simulink model "regenerative_brk_27_08"  (R2023a)
settings: Solver=VariableStepAuto  StartTime=0.0  StopTime=10.0  RelTol=1e-3
undefined symbols (not defined in the file): Ion, Lithium, Regen_brkg_Bat_SOC_lowr_tshld, Regen_brkg_Bat_SOC_upp_tshld, Regen_brkg_Bat_temp_lowr_tshld, Regen_brkg_Bat_temp_uppr_tshld, Regen_brkg_Bat_vtg_lowr_tshld, Regen_brkg_Bat_vtg_uppr_tshld, Regen_brkg_Brk_Frce_uppr_tshld, Regen_brkg_hall_sensr_vtg_lowr_tshld, Regen_brkg_Inverter_crnt_uppr_tshld, Regen_brkg_Motor_crnt_uppr_tshld, Regen_brkg_Motor_OFF_tshld, Regen_brkg_Motor_ON_tshld, Regen_brkg_Motor_spd_tshld, Regen_brkg_Motor_temp_uppr_tshld, Regen_brkg_spr_cap_temp_uppr_tshld, Regen_brkg_spr_cap_vtg_uppr_tshld, Regen_brkg_system_crnt_lowr_tshld, Regen_brkg_system_crnt_uppr_tshld, Regen_brkg_vhcl_ignition_status_OFF, Regen_brkg_vhcl_ignition_status_ON, Regen_brkg_vhcl_spd_lowr_tshld
libraries: simulink x8, spsMosfetLib x6, spsVoltageMeasurementLib x3, spsBatteryLib x1, spsPermanentMagnetSynchronousMachineLib x1, slpidlib x1
settings Model: DataDictionary=RGB_DataDictionary.sldd  Creator=lenovo  LastModifiedBy=Dell

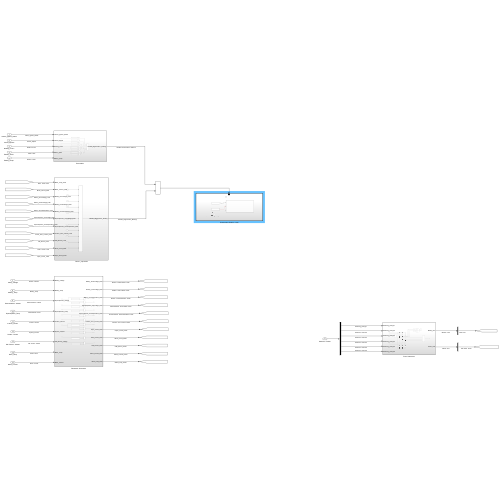
[thumbnail: Simulink's stored preview of the top-level diagram]
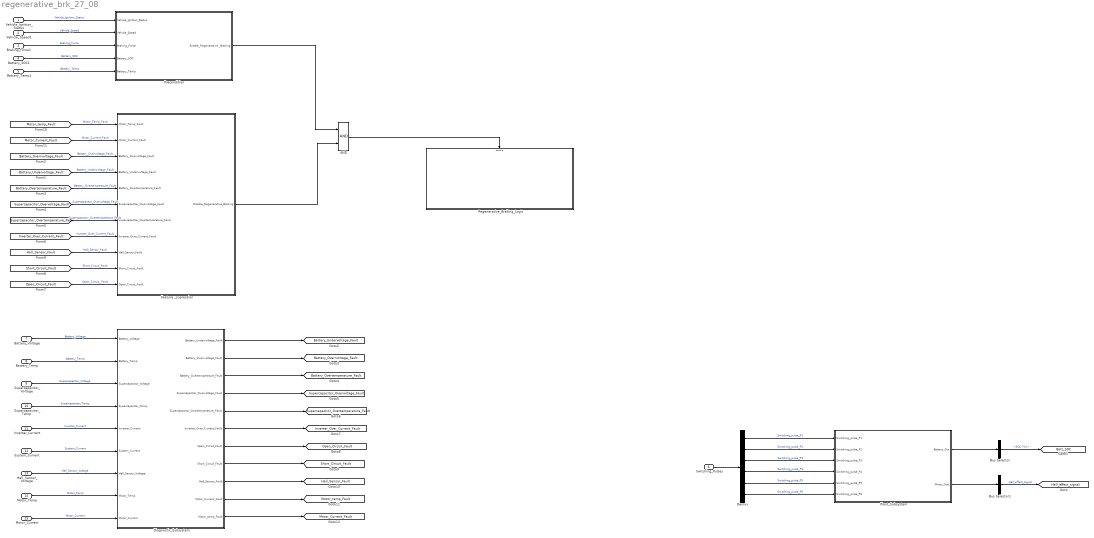
== system regenerative_brk_27_08 ==
  Vehicle_Ignition_Status : Inport
  Vehicle_Speed1 : Inport  Port=2
  Braking_Force1 : Inport  Port=3
  Battery_SOC1 : Inport  Port=4
  Battery_Temp1 : Inport  Port=5
  Switching_Pulses : Inport  Port=6
  Battery_Voltage : Inport  Port=7
  Battery_Temp : Inport  Port=8
  Supercapacitor_Voltage : Inport  Port=9
  Supercapacitor_Temp : Inport  Port=10
  Inverter_Current : Inport  Port=11
  System_Current : Inport  Port=12
  Hall_Sensor_Voltage : Inport  Port=13
  Motor_Temp : Inport  Port=14
  Motor_Current : Inport  Port=15
  AND : Logic  AllPortsSameDT=off  OutDataTypeStr=boolean
  Bus Selector : BusSelector  OutputSignals=SOC (%)
  Bus Selector1 : BusSelector  OutputSignals=Hall effect signal h_a,Hall effect signal h_b,Hall effect signal h_c  OutputAsBus=on
  Demux : Demux  Outputs=6
  Diagnostic_Subsystem : Subsystem
  Feature _supression : Subsystem
  Plant_Subsystem : Subsystem
  Precondition : Subsystem
  Regenerative_Braking_Logic : Subsystem  TreatAsAtomicUnit=on
  tag scope: Batt_SOC=global, Battery_Overrvoltage_Fault=global, Battery_Overtemperature_Fault=global, Battery_Undervoltage_Fault=global, Hall_Sensor_Fault=global, Hall_effect_signal=global, Inverter_Over_Current_Fault=global, Motor_Current_Fault=global, Motor_temp_Fault=global, Open_Circuit_Fault=global, Short_Circuit_Fault=global, Supercapacitor_Overtemperature_Fault=global, Supercapacitor_Overvoltage_Fault=global
  wires:
  [Motor_temp_Fault] -> Feature _supression/1(Motor_Temp_Fault)  "Motor_Temp_Fault"
  Feature _supression/1(Disable_Regenerative_Braking) -> AND/2
  Battery_Temp1/1 -> Precondition/5(Battery_Temp)  "Battery_Temp"
  Vehicle_Speed1/1 -> Precondition/2(Vehicle_Speed)  "Vehicle_Speed"
  Precondition/1(Enable_Regenerative _Braking) -> AND/1
  Braking_Force1/1 -> Precondition/3(Braking_Force)  "Braking_Force"
  Vehicle_Ignition_Status/1 -> Precondition/1(Vehicle_Ignition_Status)  "Vehicle_Ignition_Status"
  Battery_SOC1/1 -> Precondition/4(Battery_SOC)  "Battery_SOC"
  [Inverter_Over_Current_Fault] -> Feature _supression/8("Inverter_Over_Current_Fault ")  "Inverter_Over_Current_Fault"
  [Short_Circuit_Fault] -> Feature _supression/10(Short_Circuit_Fault)  "Short_Circuit_Fault"
  [Supercapacitor_Overvoltage_Fault] -> Feature _supression/6(Supercapacitor_Overvoltage_Fault)  "Supercapacitor_Overvoltage_Fault"
  [Battery_Overtemperature_Fault] -> Feature _supression/5(Battery_Overtemperature_Fault)  "Battery_Overtemperature_Fault"
  [Supercapacitor_Overtemperature_Fault] -> Feature _supression/7(Supercapacitor_Overtemperature_Fault)  "Supercapacitor_Overtemperature_Fault"
  [Open_Circuit_Fault] -> Feature _supression/11(Open_Circuit_Fault)  "Open_Circuit_ Fault"
  [Battery_Undervoltage_Fault] -> Feature _supression/4(Battery_Undervoltage_Fault)  "Battery_Undervoltage_Fault"
  [Hall_Sensor_Fault] -> Feature _supression/9(Hall_Sensor_Fault)  "Hall_Sensor_Fault"
  [Motor_Current_Fault] -> Feature _supression/2(Motor_Current_Fault)  "Motor_Current_Fault"
  Bus Selector/1 -> [Batt_SOC]  "<SOC (%)>"
  Demux/1 -> Plant_Subsystem/1(Switching_pulse_P1)  "Switching_pulse_P1"
  Demux/3 -> Plant_Subsystem/3(Switching_pulse_P3)  "Switching_pulse_P3"
  Demux/5 -> Plant_Subsystem/5(Switching_pulse_P5)  "Switching_pulse_P5"
  Demux/6 -> Plant_Subsystem/6(Switching_pulse_P6)  "Switching_pulse_P6"
  Demux/2 -> Plant_Subsystem/2(Switching_pulse_P2)  "Switching_pulse_P2"
  Switching_Pulses/1 -> Demux/1
  Demux/4 -> Plant_Subsystem/4(Switching_pulse_P4)  "Switching_pulse_P4"
  Plant_Subsystem/1(Battery_Out) -> Bus Selector/1
  Bus Selector1/1 -> [Hall_effect_signal]  "Hall_effect_signal"
  Plant_Subsystem/2(Motor_Outt) -> Bus Selector1/1
  Motor_Current/1 -> Diagnostic_Subsystem/9(Motor_Current)  "Motor_Current"
  Motor_Temp/1 -> Diagnostic_Subsystem/8(Motor_Temp)  "Motor_Temp"
  Inverter_Current/1 -> Diagnostic_Subsystem/5(Inverter_Current)  "Inverter_Current"
  Supercapacitor_Temp/1 -> Diagnostic_Subsystem/4(Supercapacitor_Temp)  "Supercapacitor_Temp"
  Battery_Temp/1 -> Diagnostic_Subsystem/2(Battery_Temp)  "Battery_Temp"
  Hall_Sensor_Voltage/1 -> Diagnostic_Subsystem/7(Hall_Sensor_Voltage)  "Hall_Sensor_Voltage"
  Supercapacitor_Voltage/1 -> Diagnostic_Subsystem/3(Supercapacitor_Voltage)  "Supercapacitor_Voltage"
  Battery_Voltage/1 -> Diagnostic_Subsystem/1(Battery_Voltage)  "Battery_Voltage"
  System_Current/1 -> Diagnostic_Subsystem/6(System_Current)  "System_Current"
  Diagnostic_Subsystem/11(Motor_temp_Fault) -> [Motor_Current_Fault]
  Diagnostic_Subsystem/9(Hall_Sensor_Fault) -> [Hall_Sensor_Fault]
  Diagnostic_Subsystem/10(Motor_Current_Fault) -> [Motor_temp_Fault]
  Diagnostic_Subsystem/8(Short_Circuit_Fault) -> [Short_Circuit_Fault]
  Diagnostic_Subsystem/4(Supercapacitor_Overvoltage_Fault) -> [Supercapacitor_Overvoltage_Fault]
  Diagnostic_Subsystem/6(Inverter_Over_Current_Fault) -> [Inverter_Over_Current_Fault]
  Diagnostic_Subsystem/1(Battery_Undervoltage_Fault) -> [Battery_Undervoltage_Fault]
  Diagnostic_Subsystem/3(Battery_Overtemperature_Fault) -> [Battery_Overtemperature_Fault]
  Diagnostic_Subsystem/5(Supercapacitor_Overtemperature_Fault) -> [Supercapacitor_Overtemperature_Fault]
  Diagnostic_Subsystem/7(Open_Circuit_Fault) -> [Open_Circuit_Fault]
  Diagnostic_Subsystem/2(Battery_Overrvoltage_Fault) -> [Battery_Overrvoltage_Fault]
  [Battery_Overrvoltage_Fault] -> Feature _supression/3(Battery_Overvoltage_Fault)  "Battery_Overvoltage_Fault"
  AND/1 -> Regenerative_Braking_Logic/Enable

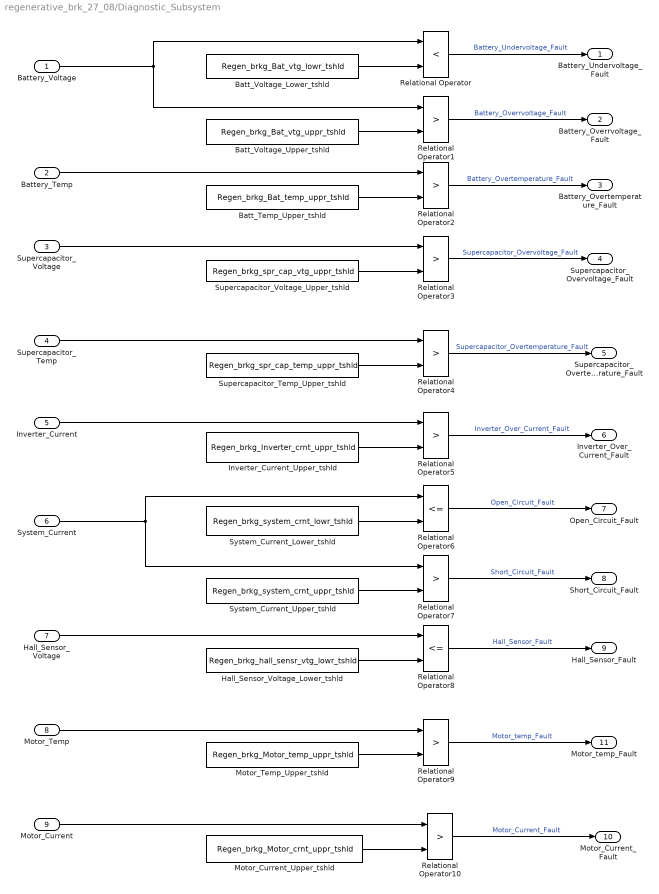
== system regenerative_brk_27_08/Diagnostic_Subsystem ==
  Battery_Voltage : Inport
  Battery_Temp : Inport  Port=2
  Supercapacitor_Voltage : Inport  Port=3
  Supercapacitor_Temp : Inport  Port=4
  Inverter_Current : Inport  Port=5
  System_Current : Inport  Port=6
  Hall_Sensor_Voltage : Inport  Port=7
  Motor_Temp : Inport  Port=8
  Motor_Current : Inport  Port=9
  "Batt_Temp_Upper_tshld  " : Constant  Value=Regen_brkg_Bat_temp_uppr_tshld
  "Batt_Voltage_Lower_tshld  " : Constant  Value=Regen_brkg_Bat_vtg_lowr_tshld
  "Batt_Voltage_Upper_tshld  " : Constant  Value=Regen_brkg_Bat_vtg_uppr_tshld
  "Hall_Sensor_Voltage_Lower_tshld  " : Constant  Value=Regen_brkg_hall_sensr_vtg_lowr_tshld
  "Inverter_Current_Upper_tshld  " : Constant  Value=Regen_brkg_Inverter_crnt_uppr_tshld
  "Motor_Current_Upper_tshld " : Constant  Value=Regen_brkg_Motor_crnt_uppr_tshld
  "Motor_Temp_Upper_tshld  " : Constant  Value=Regen_brkg_Motor_temp_uppr_tshld
  Relational Operator : RelationalOperator  Operator=<  OutDataTypeStr=boolean  RndMeth=Simplest  InputSameDT=off
  Relational Operator{1..5,7,9..10} (8 alike) : RelationalOperator  Operator=>  OutDataTypeStr=boolean  RndMeth=Simplest  InputSameDT=off
  Relational Operator6 : RelationalOperator  Operator=<=  OutDataTypeStr=boolean  RndMeth=Simplest  InputSameDT=off
  Relational Operator8 : RelationalOperator  Operator=<=  OutDataTypeStr=boolean  RndMeth=Simplest  InputSameDT=off
  "Supercapacitor_Temp_Upper_tshld  " : Constant  Value=Regen_brkg_spr_cap_temp_uppr_tshld
  "Supercapacitor_Voltage_Upper_tshld  " : Constant  Value=Regen_brkg_spr_cap_vtg_uppr_tshld
  "System_Current_Lower_tshld  " : Constant  Value=Regen_brkg_system_crnt_lowr_tshld
  "System_Current_Upper_tshld  " : Constant  Value=Regen_brkg_system_crnt_uppr_tshld
  Battery_Undervoltage_Fault : Outport
  Battery_Overrvoltage_Fault : Outport  Port=2
  Battery_Overtemperature_Fault : Outport  Port=3
  Supercapacitor_Overvoltage_Fault : Outport  Port=4
  Supercapacitor_Overtemperature_Fault : Outport  Port=5
  Inverter_Over_Current_Fault : Outport  Port=6
  Open_Circuit_Fault : Outport  Port=7
  Short_Circuit_Fault : Outport  Port=8
  Hall_Sensor_Fault : Outport  Port=9
  Motor_Current_Fault : Outport  Port=10
  Motor_temp_Fault : Outport  Port=11
  wires:
  "Batt_Voltage_Lower_tshld  "/1 -> Relational Operator/2
  Battery_Voltage/1 -> Relational Operator1/1, Relational Operator/1
  "Batt_Voltage_Upper_tshld  "/1 -> Relational Operator1/2
  Relational Operator/1 -> Battery_Undervoltage_Fault/1  "Battery_Undervoltage_Fault"
  Battery_Temp/1 -> Relational Operator2/1
  "Batt_Temp_Upper_tshld  "/1 -> Relational Operator2/2
  Relational Operator2/1 -> Battery_Overtemperature_Fault/1  "Battery_Overtemperature_Fault"
  Relational Operator1/1 -> Battery_Overrvoltage_Fault/1  "Battery_Overrvoltage_Fault"
  Supercapacitor_Voltage/1 -> Relational Operator3/1
  "Supercapacitor_Voltage_Upper_tshld  "/1 -> Relational Operator3/2
  Relational Operator3/1 -> Supercapacitor_Overvoltage_Fault/1  "Supercapacitor_Overvoltage_Fault"
  "Supercapacitor_Temp_Upper_tshld  "/1 -> Relational Operator4/2
  Relational Operator4/1 -> Supercapacitor_Overtemperature_Fault/1  "Supercapacitor_Overtemperature_Fault"
  Supercapacitor_Temp/1 -> Relational Operator4/1
  Inverter_Current/1 -> Relational Operator5/1
  "Inverter_Current_Upper_tshld  "/1 -> Relational Operator5/2
  Relational Operator5/1 -> Inverter_Over_Current_Fault/1  "Inverter_Over_Current_Fault"
  Relational Operator6/1 -> Open_Circuit_Fault/1  "Open_Circuit_Fault"
  "System_Current_Lower_tshld  "/1 -> Relational Operator6/2
  System_Current/1 -> Relational Operator7/1, Relational Operator6/1
  "System_Current_Upper_tshld  "/1 -> Relational Operator7/2
  Relational Operator7/1 -> Short_Circuit_Fault/1  "Short_Circuit_Fault"
  Hall_Sensor_Voltage/1 -> Relational Operator8/1
  "Hall_Sensor_Voltage_Lower_tshld  "/1 -> Relational Operator8/2
  Relational Operator8/1 -> Hall_Sensor_Fault/1  "Hall_Sensor_Fault"
  "Motor_Current_Upper_tshld "/1 -> Relational Operator10/2
  Relational Operator10/1 -> Motor_Current_Fault/1  "Motor_Current_Fault"
  Motor_Current/1 -> Relational Operator10/1
  Relational Operator9/1 -> Motor_temp_Fault/1  "Motor_temp_Fault"
  Motor_Temp/1 -> Relational Operator9/1
  "Motor_Temp_Upper_tshld  "/1 -> Relational Operator9/2

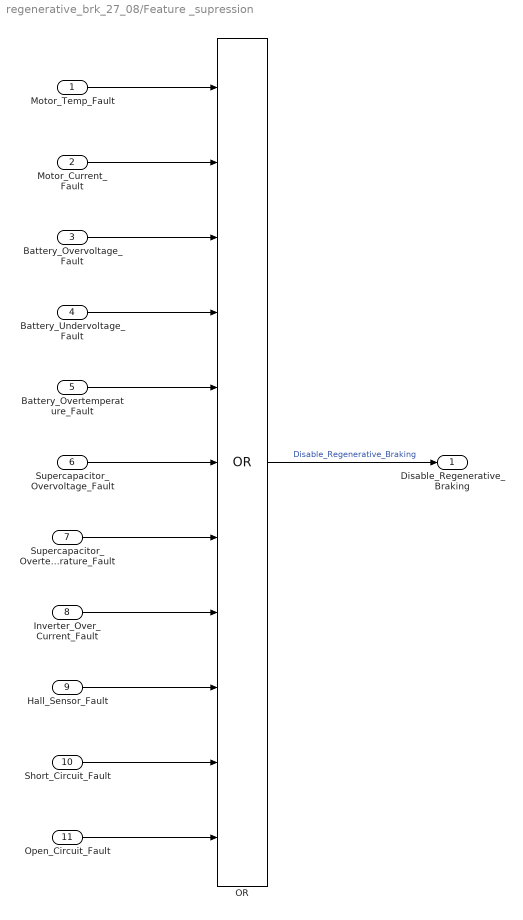
== system regenerative_brk_27_08/Feature _supression ==
  Motor_Temp_Fault : Inport
  Motor_Current_Fault : Inport  Port=2
  Battery_Overvoltage_Fault : Inport  Port=3
  Battery_Undervoltage_Fault : Inport  Port=4
  Battery_Overtemperature_Fault : Inport  Port=5
  Supercapacitor_Overvoltage_Fault : Inport  Port=6
  Supercapacitor_Overtemperature_Fault : Inport  Port=7
  "Inverter_Over_Current_Fault " : Inport  Port=8
  Hall_Sensor_Fault : Inport  Port=9
  Short_Circuit_Fault : Inport  Port=10
  Open_Circuit_Fault : Inport  Port=11
  OR : Logic  Operator=OR  Inputs=11  AllPortsSameDT=off  OutDataTypeStr=boolean
  Disable_Regenerative_Braking : Outport
  wires:
  Motor_Temp_Fault/1 -> OR/1
  OR/1 -> Disable_Regenerative_Braking/1  "Disable_Regenerative_Braking"
  Battery_Overvoltage_Fault/1 -> OR/3
  Battery_Undervoltage_Fault/1 -> OR/4
  Battery_Overtemperature_Fault/1 -> OR/5
  Supercapacitor_Overvoltage_Fault/1 -> OR/6
  Supercapacitor_Overtemperature_Fault/1 -> OR/7
  "Inverter_Over_Current_Fault "/1 -> OR/8
  Hall_Sensor_Fault/1 -> OR/9
  Short_Circuit_Fault/1 -> OR/10
  Open_Circuit_Fault/1 -> OR/11
  Motor_Current_Fault/1 -> OR/2

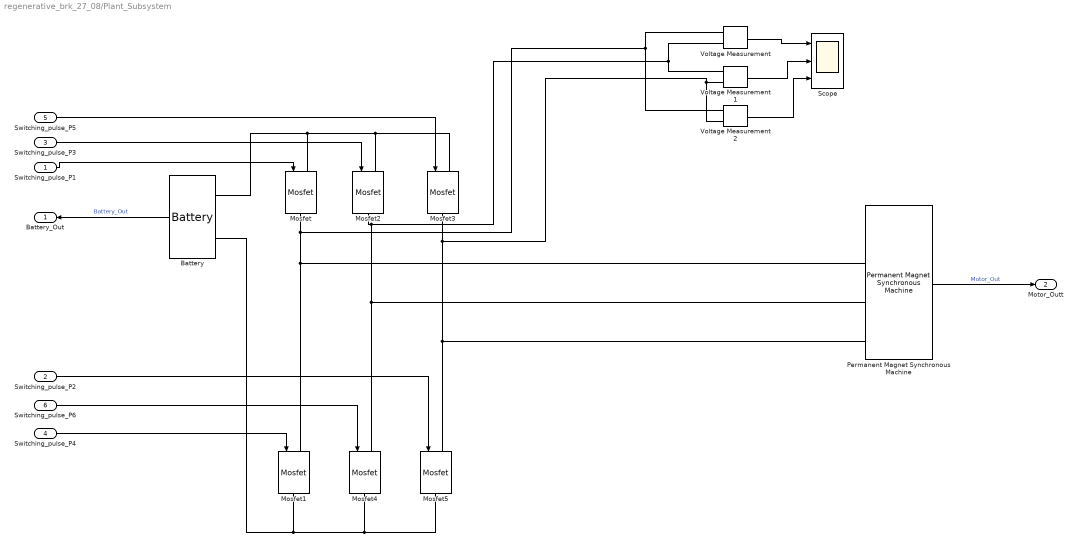
== system regenerative_brk_27_08/Plant_Subsystem ==
  Switching_pulse_P1 : Inport
  Switching_pulse_P2 : Inport  Port=2
  Switching_pulse_P3 : Inport  Port=3
  Switching_pulse_P4 : Inport  Port=4
  Switching_pulse_P5 : Inport  Port=5
  Switching_pulse_P6 : Inport  Port=6
  Battery : spsBatteryLib/Battery  BatType=Lithium-Ion  ShowTempParam=off  ThermalPreset=no  ShowAgeParam=off  NomV=300  NomQ=50  SOC=50  Batt_Tr=30  PresetModel=on  MaxQ=50  MinV=225  FullV=349.1961  Dis_rate=21.7391  R=0.06  Normal_OP=45.2174  expZone="[324.1158      2.456522]"  current=[6.5 13 32.5]  Units=Time  Tci=20  NomT=20  T2=-30  MaxQ2=4.8  FullV2=7.1  Normal_OP2=5.655  expZone2="[6.58           1]"  Rca=0.6  ti=2000  Dp=0  Neq0=0  Tsim=1e6  Ta1=25  Qeol=5.4*0.9  Reol=0.013333*1.2  Char_age=[2.3478, 3]  Dis_age=[2.3478, 10]  N1=1500  N2=10500  N3=1000  N4=1400  Ta2=45  N5=950
  Mosfet{,1..5} (6 alike) : spsMosfetLib/Mosfet  Ron=0.1  Lon=0  Rd=0.01  Vfd=0  IC=0  Rs=1e5  Cs=inf  Measurements=off
  Permanent Magnet Synchronous Machine : spsPermanentMagnetSynchronousMachineLib/Permanent Magnet Synchronous Machine  NbPhases=3  FluxDistribution=Sinusoidal  RotorType=Round  MechanicalLoad=Torque Tm  PresetModel=No  ShowDetailedParameters=on  MeasurementBus=off  Resistance=0.0485  Inductance=8.5e-3  dqInductances=[8.5e-3,8.5e-3]  La=0.000395  MachineConstant=Flux linkage established by magnets (V.s)  Flux=0.1194  VoltageCst=86.6271  TorqueCst=0.7164  Flat=120  Mechanical=[0.0027 0.0004924 4 0]  PolePairs=4  InitialConditions=[0,0, 0,0]  InitialConditions5ph=[0 0 0 0 0 0]  RefAngle=90 degrees behind phase A axis (modified Park)  IterativeDiscreteModel=Trapezoidal non iterative  TsBlock=-1  TsPowergui=0
  Scope : Scope  NumInputPorts=3
  Voltage Measurement : spsVoltageMeasurementLib/Voltage Measurement  PhasorSimulation=off  OutputType=Complex  PSBequivalent=0
  Voltage Measurement1 : spsVoltageMeasurementLib/Voltage Measurement  PhasorSimulation=off  OutputType=Complex  PSBequivalent=0
  Voltage Measurement2 : spsVoltageMeasurementLib/Voltage Measurement  PhasorSimulation=off  OutputType=Complex  PSBequivalent=0
  Battery_Out : Outport
  Motor_Outt : Outport  Port=2
  wires:
  Voltage Measurement2/1 -> Scope/3
  Voltage Measurement/1 -> Scope/1
  Battery/1 -> Battery_Out/1  "Battery_Out"
  Voltage Measurement1/1 -> Scope/2
  Switching_pulse_P6/1 -> Mosfet4/1
  Switching_pulse_P2/1 -> Mosfet5/1
  Switching_pulse_P1/1 -> Mosfet/1
  Switching_pulse_P5/1 -> Mosfet3/1
  Switching_pulse_P3/1 -> Mosfet2/1
  Switching_pulse_P4/1 -> Mosfet1/1
  Permanent Magnet Synchronous Machine/1 -> Motor_Outt/1  "Motor_Out"
  connections:
  Voltage Measurement/LConn1 -- Mosfet1/LConn1 -- Permanent Magnet Synchronous Machine/LConn1 -- Mosfet/RConn1 -- Voltage Measurement2/LConn1
  Mosfet1/RConn1 -- Battery/LConn2 -- Mosfet4/RConn1 -- Mosfet5/RConn1
  Mosfet2/LConn1 -- Mosfet3/LConn1 -- Mosfet/LConn1 -- Battery/LConn1
  Mosfet2/RConn1 -- Voltage Measurement/LConn2 -- Voltage Measurement1/LConn1 -- Permanent Magnet Synchronous Machine/LConn2 -- Mosfet4/LConn1
  Mosfet3/RConn1 -- Voltage Measurement2/LConn2 -- Voltage Measurement1/LConn2 -- Mosfet5/LConn1 -- Permanent Magnet Synchronous Machine/LConn3

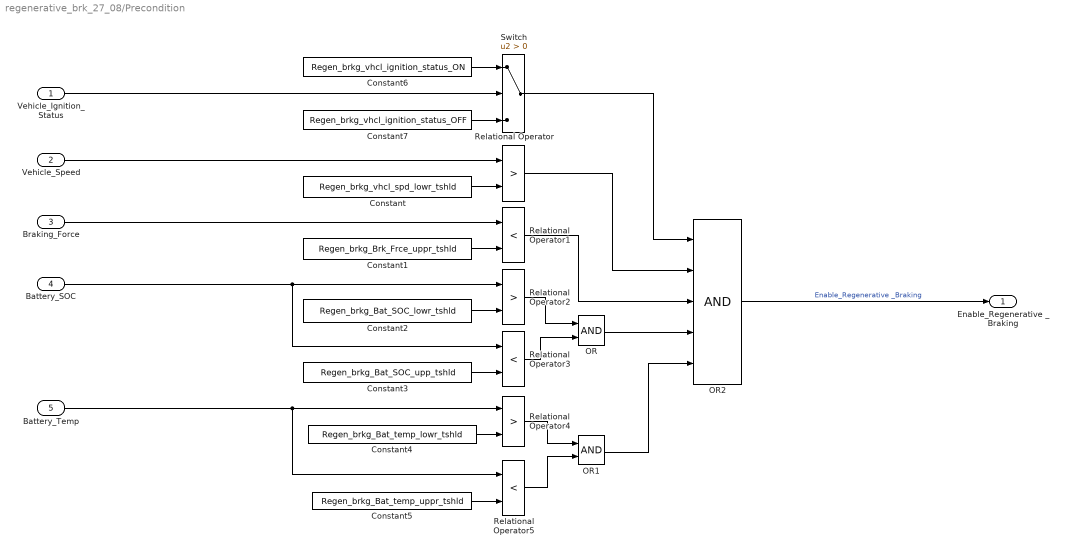
== system regenerative_brk_27_08/Precondition ==
  Vehicle_Ignition_Status : Inport
  Vehicle_Speed : Inport  Port=2
  Braking_Force : Inport  Port=3
  Battery_SOC : Inport  Port=4
  Battery_Temp : Inport  Port=5
  Constant : Constant  Value=Regen_brkg_vhcl_spd_lowr_tshld
  Constant1 : Constant  Value=Regen_brkg_Brk_Frce_uppr_tshld
  Constant2 : Constant  Value=Regen_brkg_Bat_SOC_lowr_tshld
  Constant3 : Constant  Value=Regen_brkg_Bat_SOC_upp_tshld
  Constant4 : Constant  Value=Regen_brkg_Bat_temp_lowr_tshld
  Constant5 : Constant  Value=Regen_brkg_Bat_temp_uppr_tshld
  Constant6 : Constant  Value=Regen_brkg_vhcl_ignition_status_ON
  Constant7 : Constant  Value=Regen_brkg_vhcl_ignition_status_OFF
  OR : Logic  AllPortsSameDT=off  OutDataTypeStr=boolean
  OR1 : Logic  AllPortsSameDT=off  OutDataTypeStr=boolean
  OR2 : Logic  Inputs=5  AllPortsSameDT=off  OutDataTypeStr=boolean
  Relational Operator : RelationalOperator  Operator=>  OutDataTypeStr=boolean  RndMeth=Simplest  InputSameDT=off
  Relational Operator1 : RelationalOperator  Operator=<  OutDataTypeStr=boolean  RndMeth=Simplest  InputSameDT=off
  Relational Operator2 : RelationalOperator  Operator=>  OutDataTypeStr=boolean  RndMeth=Simplest  InputSameDT=off
  Relational Operator3 : RelationalOperator  Operator=<  OutDataTypeStr=boolean  RndMeth=Simplest  InputSameDT=off
  Relational Operator4 : RelationalOperator  Operator=>  OutDataTypeStr=boolean  RndMeth=Simplest  InputSameDT=off
  Relational Operator5 : RelationalOperator  Operator=<  OutDataTypeStr=boolean  RndMeth=Simplest  InputSameDT=off
  Switch : Switch  Criteria=u2 > Threshold  SaturateOnIntegerOverflow=off  InputSameDT=off
  Enable_Regenerative _Braking : Outport
  wires:
  OR1/1 -> OR2/5
  Battery_SOC/1 -> Relational Operator2/1, Relational Operator3/1
  Constant1/1 -> Relational Operator1/2
  Battery_Temp/1 -> Relational Operator4/1, Relational Operator5/1
  Braking_Force/1 -> Relational Operator1/1
  Vehicle_Speed/1 -> Relational Operator/1
  Relational Operator3/1 -> OR/2
  Constant4/1 -> Relational Operator4/2
  Relational Operator5/1 -> OR1/2
  Relational Operator1/1 -> OR2/3
  Constant/1 -> Relational Operator/2
  Constant5/1 -> Relational Operator5/2
  Relational Operator2/1 -> OR/1
  Relational Operator4/1 -> OR1/1
  Constant3/1 -> Relational Operator3/2
  Relational Operator/1 -> OR2/2
  Constant2/1 -> Relational Operator2/2
  Constant7/1 -> Switch/3
  Constant6/1 -> Switch/1
  Vehicle_Ignition_Status/1 -> Switch/2
  OR2/1 -> Enable_Regenerative _Braking/1  "Enable_Regenerative _Braking"
  Switch/1 -> OR2/1
  OR/1 -> OR2/4

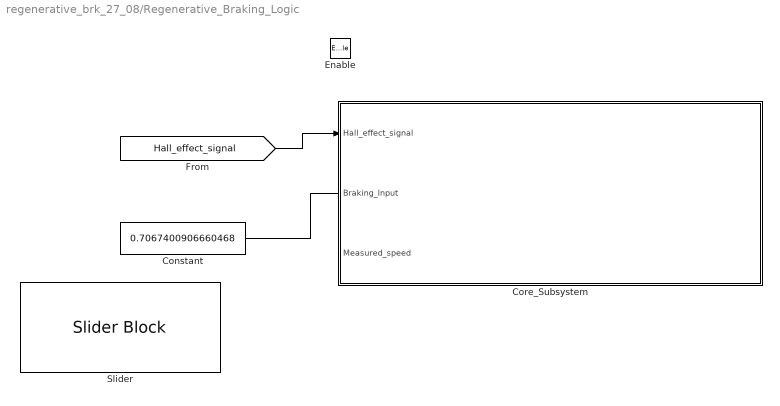
== system regenerative_brk_27_08/Regenerative_Braking_Logic ==
  Enable : EnablePort
  Constant : Constant  Value=0.7067400906660468
  Core_Subsystem : Subsystem
  Slider : SliderBlock  ScaleMax=0.99
  wires:
  [Hall_effect_signal] -> Core_Subsystem/1(Hall_effect_signal)
  Constant/1 -> ?

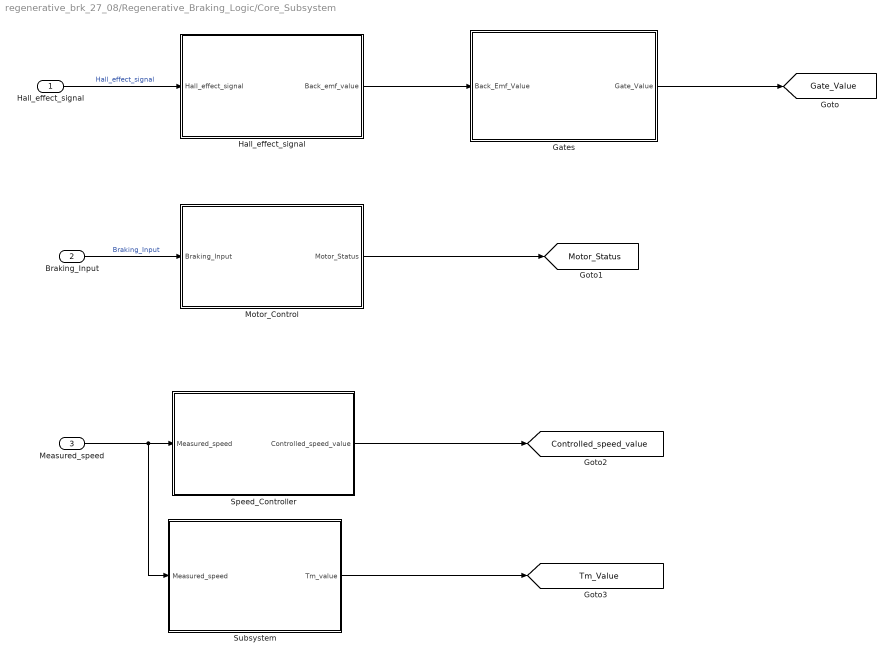
== system regenerative_brk_27_08/Regenerative_Braking_Logic/Core_Subsystem ==
  Hall_effect_signal : Inport
  Braking_Input : Inport  Port=2
  Measured_speed : Inport  Port=3
  Gates : Subsystem
  "Hall_effect_signal " : Subsystem
  Motor_Control : Subsystem
  Speed_Controller : Subsystem
  Subsystem : Subsystem
  tag scope: Controlled_speed_value=global, Gate_Value=global, Motor_Status=global, Tm_Value=global
  wires:
  Hall_effect_signal/1 -> "Hall_effect_signal "/1(Hall_effect_signal)  "Hall_effect_signal"
  "Hall_effect_signal "/1(Back_emf_value) -> Gates/1(Back_Emf_Value)
  Gates/1(Gate_Value) -> [Gate_Value]
  Subsystem/1(Tm_value) -> [Tm_Value]
  Measured_speed/1 -> Subsystem/1(Measured_speed), Speed_Controller/1(Measured_speed)
  Motor_Control/1(Motor_Status) -> [Motor_Status]
  Speed_Controller/1(Controlled_speed_value) -> [Controlled_speed_value]
  Braking_Input/1 -> Motor_Control/1(Braking_Input)  "Braking_Input"

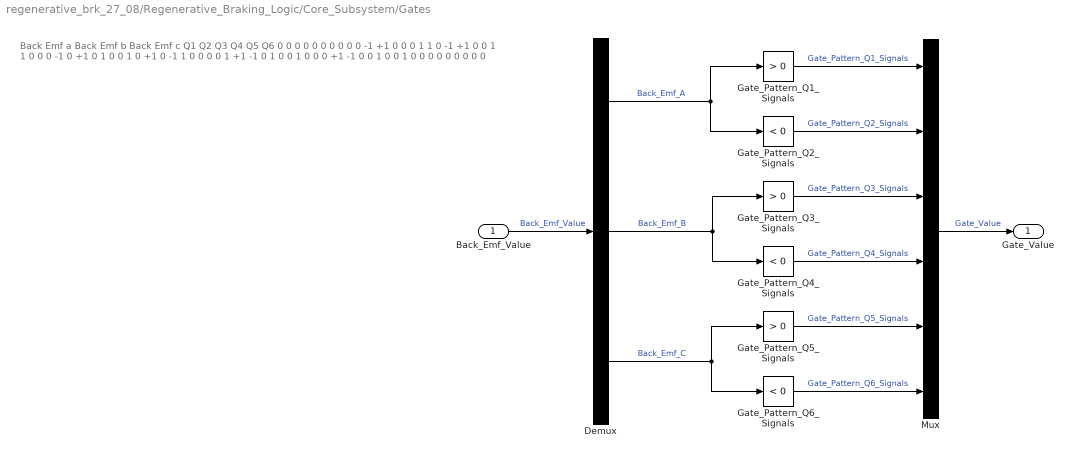
== system regenerative_brk_27_08/Regenerative_Braking_Logic/Core_Subsystem/Gates ==
  note: Back Emf a
      | Back Emf b
      | Back Emf c
      | Q1
      | Q2
      | Q3
      | Q4
      | Q5
      | Q6
      |
      | 0
      | 0
      | 0
      | 0
      | 0
      | 0
      | 0
      | 0
      | 0
      |
      | 0
      | -1
      | +1
      | 0
      | 0
      | 0
      | 1
      | 1
      | 0
      |
      | -1
      | +1
      | 0
      | 0
      | 1
      | 1
      | 0
      | 0
      | 0
      |
      | -1
      | 0
      | +1
      | 0
      | 1
      | 0
      | 0
      | 1
      | 0
      |
      | +1
      | 0
      | -1
      | 1
      | 0
      | 0
      | 0
      | 0
      | 1
      |
      | +1
      | -1
      | 0
      | 1
      | 0
      | 0
      | 1
      | 0
      | 0
      |
      | 0
      | +1
      | -1
      | 0
      | 0
      | 1
      | 0
      | 0
      | 1
      |
      | 0
      | 0
      | 0
      | 0
      | 0
      | 0
      | 0
      | 0
      | 0
  Back_Emf_Value : Inport
  Demux : Demux  Outputs=3
  Gate_Pattern_Q1_Signals : simulink/Logic and Bit Operations/Compare To Constant  relop=>  const=0  OutDataTypeStr=boolean
  Gate_Pattern_Q2_Signals : simulink/Logic and Bit Operations/Compare To Constant  relop=<  const=0  OutDataTypeStr=boolean
  Gate_Pattern_Q3_Signals : simulink/Logic and Bit Operations/Compare To Constant  relop=>  const=0  OutDataTypeStr=boolean
  Gate_Pattern_Q4_Signals : simulink/Logic and Bit Operations/Compare To Constant  relop=<  const=0  OutDataTypeStr=boolean
  Gate_Pattern_Q5_Signals : simulink/Logic and Bit Operations/Compare To Constant  relop=>  const=0  OutDataTypeStr=boolean
  Gate_Pattern_Q6_Signals : simulink/Logic and Bit Operations/Compare To Constant  relop=<  const=0  OutDataTypeStr=boolean
  Mux : Mux  Inputs=6
  Gate_Value : Outport
  wires:
  Back_Emf_Value/1 -> Demux/1  "Back_Emf_Value"
  Gate_Pattern_Q5_Signals/1 -> Mux/5  "Gate_Pattern_Q5_Signals"
  Gate_Pattern_Q2_Signals/1 -> Mux/2  "Gate_Pattern_Q2_Signals"
  Demux/1 -> Gate_Pattern_Q2_Signals/1, Gate_Pattern_Q1_Signals/1  "Back_Emf_A"
  Demux/3 -> Gate_Pattern_Q6_Signals/1, Gate_Pattern_Q5_Signals/1  "Back_Emf_C"
  Gate_Pattern_Q4_Signals/1 -> Mux/4  "Gate_Pattern_Q4_Signals"
  Demux/2 -> Gate_Pattern_Q4_Signals/1, Gate_Pattern_Q3_Signals/1  "Back_Emf_B"
  Gate_Pattern_Q6_Signals/1 -> Mux/6  "Gate_Pattern_Q6_Signals"
  Gate_Pattern_Q1_Signals/1 -> Mux/1  "Gate_Pattern_Q1_Signals"
  Mux/1 -> Gate_Value/1  "Gate_Value"
  Gate_Pattern_Q3_Signals/1 -> Mux/3  "Gate_Pattern_Q3_Signals"

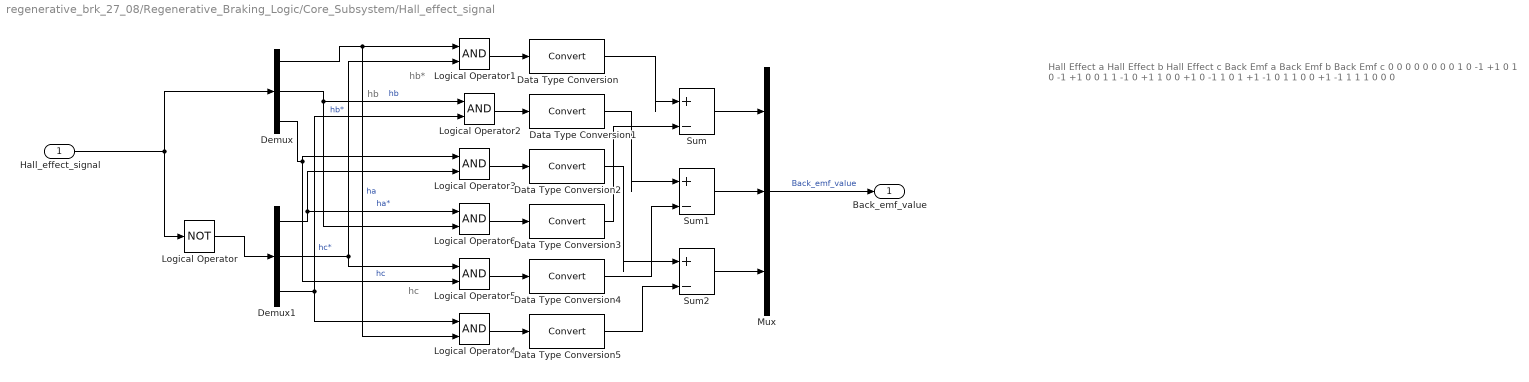
== system regenerative_brk_27_08/Regenerative_Braking_Logic/Core_Subsystem/Hall_effect_signal  ==
  note: hc
  note: hb
  note: hb*
  note: Hall Effect a
      | Hall Effect b
      | Hall Effect c
      | Back Emf a
      | Back Emf b
      | Back Emf c
      |
      | 0
      | 0
      | 0
      | 0
      | 0
      | 0
      |
      | 0
      | 0
      | 1
      | 0
      | -1
      | +1
      |
      | 0
      | 1
      | 0
      | -1
      | +1
      | 0
      |
      | 0
      | 1
      | 1
      | -1
      | 0
      | +1
      |
      | 1
      | 0
      | 0
      | +1
      | 0
      | -1
      |
      | 1
      | 0
      | 1
      | +1
      | -1
      | 0
      |
      | 1
      | 1
      | 0
      | 0
      | +1
      | -1
      |
      | 1
      | 1
      | 1
      | 0
      | 0
      | 0
  Hall_effect_signal : Inport
  Data Type Conversion{,1..5} (6 alike) : DataTypeConversion  SaturateOnIntegerOverflow=off  RndMeth=Floor
  Demux : Demux  Outputs=3
  Demux1 : Demux  Outputs=3
  Logical Operator : Logic  Operator=NOT  AllPortsSameDT=off  OutDataTypeStr=boolean
  Logical Operator{1..6} (6 alike) : Logic  AllPortsSameDT=off  OutDataTypeStr=boolean
  Mux : Mux  Inputs=3
  Sum : Sum  Inputs=|+-
  Sum1 : Sum  Inputs=|+-
  Sum2 : Sum  Inputs=|+-
  Back_emf_value : Outport
  wires:
  Hall_effect_signal/1 -> Logical Operator/1, Demux/1
  Logical Operator/1 -> Demux1/1
  Sum/1 -> Mux/1
  Sum1/1 -> Mux/2
  Sum2/1 -> Mux/3
  Logical Operator1/1 -> Data Type Conversion/1
  Logical Operator2/1 -> Data Type Conversion1/1
  Logical Operator3/1 -> Data Type Conversion2/1
  Logical Operator6/1 -> Data Type Conversion3/1
  Logical Operator5/1 -> Data Type Conversion4/1
  Logical Operator4/1 -> Data Type Conversion5/1
  Data Type Conversion/1 -> Sum/1
  Data Type Conversion3/1 -> Sum/2
  Data Type Conversion1/1 -> Sum1/1
  Data Type Conversion4/1 -> Sum1/2
  Data Type Conversion2/1 -> Sum2/1
  Data Type Conversion5/1 -> Sum2/2
  Mux/1 -> Back_emf_value/1  "Back_emf_value"
  Demux/1 -> Logical Operator4/2, Logical Operator1/1  "ha"
  Demux1/2 -> Logical Operator5/1, Logical Operator1/2  "hb*"
  Demux/2 -> Logical Operator6/2, Logical Operator2/1  "hb"
  Demux1/3 -> Logical Operator4/1, Logical Operator2/2  "hc*"
  Demux/3 -> Logical Operator5/2, Logical Operator3/1  "hc"
  Demux1/1 -> Logical Operator6/1, Logical Operator3/2  "ha*"

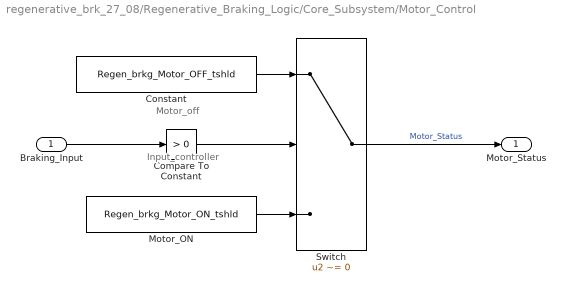
== system regenerative_brk_27_08/Regenerative_Braking_Logic/Core_Subsystem/Motor_Control ==
  note: Input_controller
  note: Motor_off
  Braking_Input : Inport
  Compare To Constant : simulink/Logic and Bit Operations/Compare To Constant  relop=>  const=0  OutDataTypeStr=boolean
  Constant : Constant  Value=Regen_brkg_Motor_OFF_tshld  OutDataTypeStr=boolean
  Motor_ON : Constant  Value=Regen_brkg_Motor_ON_tshld  OutDataTypeStr=boolean
  Switch : Switch  Criteria=u2 ~= 0  SaturateOnIntegerOverflow=off  InputSameDT=off
  Motor_Status : Outport
  wires:
  Braking_Input/1 -> Compare To Constant/1
  Compare To Constant/1 -> Switch/2
  Constant/1 -> Switch/1
  Motor_ON/1 -> Switch/3
  Switch/1 -> Motor_Status/1  "Motor_Status"

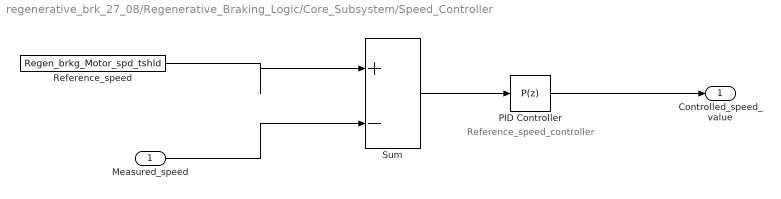
== system regenerative_brk_27_08/Regenerative_Braking_Logic/Core_Subsystem/Speed_Controller ==
  note: Reference_speed_controller
  Measured_speed : Inport
  PID Controller : slpidlib/PID Controller  Controller=P  Form=Parallel  TimeDomain=Discrete-time  UseExternalTs=off  SampleTime=-1  IntegratorMethod=Forward Euler  FilterMethod=Forward Euler  ControllerParametersSource=internal  P=0.1  I=1  UseKiTs=off  D=0  N=100  UseFilter=on  TunerSelectOption=Transfer Function Based (PID Tuner App)  InitialConditionSource=internal  InitialConditionForIntegrator=0  InitialConditionForFilter=0  DifferentiatorICPrevScaledInput=0  ExternalReset=none  TrackingMode=off  Kt=1  LimitOutput=off  SatLimitsSource=internal  UpperSaturationLimit=inf  LowerSaturationLimit=-inf  LinearizeAsGain=on  AntiWindupMode=none  Kb=1  LimitIntegrator=off  UpperIntegratorSaturationLimit=inf  LowerIntegratorSaturationLimit=-inf  POutMin=[]  POutMax=[]  IOutMin=[]  IOutMax=[]  DOutMin=[]  DOutMax=[]  NOutMin=[]  NOutMax=[]  SumOutMin=[]  SumOutMax=[]  SaturationOutMin=[]  SaturationOutMax=[]  PParamMin=[]  PParamMax=[]  IParamMin=[]  IParamMax=[]  DParamMin=[]  DParamMax=[]  NParamMin=[]  NParamMax=[]  KbParamMin=[]  KbParamMax=[]  KtParamMin=[]  KtParamMax=[]  KbOutMin=[]  KbOutMax=[]  KtOutMin=[]  KtOutMax=[]  IntegratorOutMin=[]  IntegratorOutMax=[]  FilterOutMin=[]  FilterOutMax=[]  SumI1OutMin=[]  SumI1OutMax=[]  SumI2OutMin=[]  SumI2OutMax=[]  SumI3OutMin=[]  SumI3OutMax=[]  SumI4OutMin=[]  SumI4OutMax=[]  SumDOutMin=[]  SumDOutMax=[]  DifferentiatorOutMin=[]  DifferentiatorOutMax=[]  FilterDiffOutCoefMin=[]  FilterDiffOutCoefMax=[]  ReciprocalOutMin=[]  ReciprocalOutMax=[]  SumDenOutMin=[]  SumDenOutMax=[]  SumNumOutMin=[]  SumNumOutMax=[]  DivideOutMin=[]  DivideOutMax=[]  UdiffTsProdOutMin=[]  UdiffTsProdOutMax=[]  NTsProdOutMin=[]  NTsProdOutMax=[]  UintegralTsProdOutMin=[]  UintegralTsProdOutMax=[]  UngainTsProdOutMin=[]  UngainTsProdOutMax=[]  ClampingZeroOutDataTypeStr=Inherit: Inherit via back propagation  ClampingZeroOutMin=[]  ClampingZeroOutMax=[]  FilterDenConstantOutDataTypeStr=Inherit: Inherit via back propagation  FilterDenConstantOutMin=[]  FilterDenConstantOutMax=[]  PCopyOutDataTypeStr=Inherit: Inherit via back propagation  PCopyOutMin=[]  PCopyOutMax=[]  NCopyOutDataTypeStr=Inherit: Inherit via back propagation  NCopyOutMin=[]  NCopyOutMax=[]  IntegratorContinuousStateAttributes=''  IntegratorStateMustResolveToSignalObject=off  IntegratorRTWStateStorageClass=Auto  FilterContinuousStateAttributes=''  FilterStateMustResolveToSignalObject=off  FilterRTWStateStorageClass=Auto  ParallelPVariant=InternalParameters  IdealPVariant=Disabled  IVariant=Disabled  DVariant=Disabled  IntegratorVariant=Disabled  SatVariant=Disabled  AWVariant=Disabled  PCopyVariant=Disabled  TRVariant=Disabled  FdbkBlocksVariant=Forward  IdealPFdbkVariant=Disabled  SatFdbkVariant=Disabled  DerivativeFilterVariant=Disabled  NVariant=Disabled  NCopyVariant=Disabled_SignalSpec  FilterICVariant=Disabled  IntegratorICVariant=Disabled  ExternalResetVariant=Disabled  TRSumVariant=Passthrough  SumFdbkVariant=Disabled  SumVariant=Passthrough_P  TsampFilterVariant=InternalTs  TsampNgainVariant=Passthrough  TsampIntegralVariant=Disabled_SignalSpec  ExternalSaturationOutDataTypeStr=Inherit: Same as second input
  Reference_speed : Constant  Value=Regen_brkg_Motor_spd_tshld
  Sum : Sum  Inputs=|+-
  Controlled_speed_value : Outport
  wires:
  Measured_speed/1 -> Sum/2
  Reference_speed/1 -> Sum/1
  Sum/1 -> PID Controller/1
  PID Controller/1 -> Controlled_speed_value/1

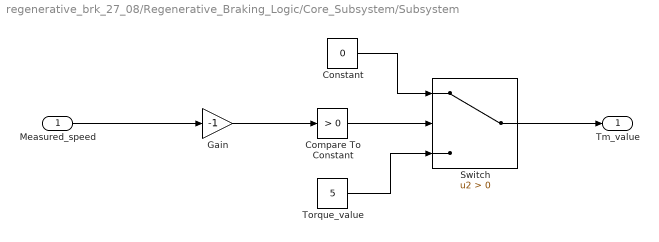
== system regenerative_brk_27_08/Regenerative_Braking_Logic/Core_Subsystem/Subsystem ==
  Measured_speed : Inport
  Compare To Constant : simulink/Logic and Bit Operations/Compare To Constant  relop=>  const=0  OutDataTypeStr=boolean
  Constant : Constant  Value=0
  Gain : Gain  Gain=-1
  Switch : Switch  Criteria=u2 > Threshold  SaturateOnIntegerOverflow=off  InputSameDT=off
  Torque_value : Constant  Value=5
  Tm_value : Outport
  wires:
  Measured_speed/1 -> Gain/1
  Gain/1 -> Compare To Constant/1
  Constant/1 -> Switch/1
  Compare To Constant/1 -> Switch/2
  Torque_value/1 -> Switch/3
  Switch/1 -> Tm_value/1
